simulink model "zad_1"  (R2023b)
settings: Solver=VariableStepAuto  StartTime=0.0  StopTime=20  RelTol=1e-3
settings Model: Creator=Asus  LastModifiedBy=Asus

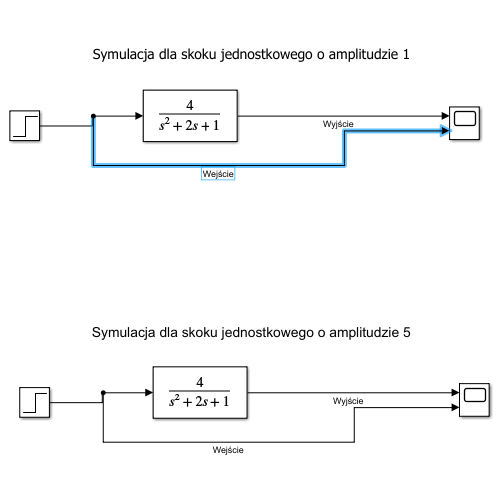
[thumbnail: Simulink's stored preview of the top-level diagram]
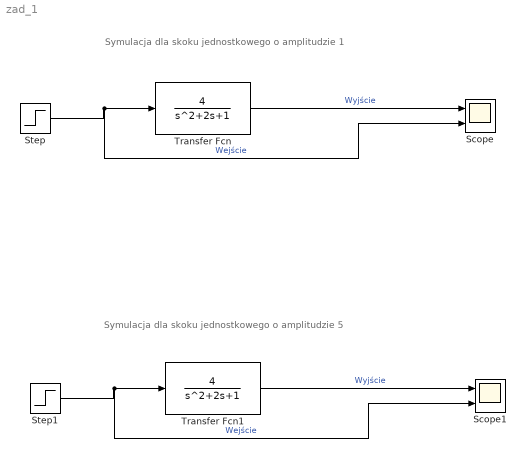
== system zad_1 ==
  note: Symulacja dla skoku jednostkowego o amplitudzie 1
  note: Symulacja dla skoku jednostkowego o amplitudzie 5
  Scope : Scope  NumInputPorts=2
  Scope1 : Scope  NumInputPorts=2
  Step : Step  Time=3  SampleTime=0
  Step1 : Step  Time=3  After=5  SampleTime=0
  Transfer Fcn : TransferFcn  Numerator=[4]
  Transfer Fcn1 : TransferFcn  Numerator=[4]
  wires:
  Step/1 -> Scope/2, Transfer Fcn/1  "Wejście"
  Transfer Fcn/1 -> Scope/1  "Wyjście"
  Step1/1 -> Scope1/2, Transfer Fcn1/1  "Wejście"
  Transfer Fcn1/1 -> Scope1/1  "Wyjście"
